simulink model "Model_GBXCluctchOpt_V5"  (R2024b)
settings: Solver=VariableStepAuto  StartTime=0.0  StopTime=552  RelTol=1e-5
undefined symbols (not defined in the file): Bdy_facCoG_C, Bdy_facTireFric_C, Bdy_lenRadiusWheel_C, Bdy_lenWheelBase_C, Bdy_lenZCoG_C, Bdy_mEquivalentJ_C, Bdy_mVeh_C, Bdy_vsqr2frc_C, Drv_kmh2gradtqDriver_C, Drv_kmh2tqDriver_C, Edr_pwr_LossMap_AXIS, Edr_pwrInverterLosses_MAP, Edr_pwrMachineLosses_MAP, Edr_rpm_InvLossMap_AXIS, Edr_rpm_MachLossMap_AXIS, Edr_rpm_MaxMinTq_AXIS, Edr_rpmMax_C, Edr_tq_MachLossMap_AXIS, Edr_tqEffMax_CUR, Env_facSlope_WLTC_CUR, Env_facSlopeBAB185_CUR, Env_facSlopeCrossCountry_CUR, Env_kmhDesBAB185_CUR, Env_kmhDesCrossCountry_CUR, Env_vVehDes_NEDC_kmh, Env_vVehDes_WLTC_kmh, Env_vVehTime_NEDC_s, Env_vVehTime_WLTC_s, Gbx_facGbxRatioRe_C, Ice_derfacLoadDecrease_MAP, Ice_derfacLoadIncrease_MAP, Ice_etaLam_CUR, Ice_facEtaCocMax_MAP, Ice_facFuelEnRich_MAP, Ice_KUMSRL_C, Ice_Lambda_AXIS, Ice_relLoad2relTqOptIgnLamOne_MAP, Ice_relLoad_AXIS, Ice_relLoad_LoadDyn_AXIS, Ice_relLoad_Max_CUR, Ice_relTq_AXIS, Ice_relTqInr2TqInr_C, Ice_relTqOptIgnLamOne2relLoad_MAP, Ice_rpm_AXIS, Ice_rpm_LoadDyn_AXIS, Ice_rpm_relLoadMax_AXIS, Ice_tqLossesIce_MAP, Pnt_capBat_C, Pnt_facSocBatOcv_AXIS, Pnt_facSocInit_C, Pnt_iBatChrgMax_C, Pnt_iBatDisChrgMax_C, Pnt_resBatInner_C, Pnt_uBatMax_C, Pnt_uBatMin_C, Pnt_uBatOcv_CUR, Vco_flgEdrExists_CFG, Vco_flgIceCluAlwClosed_CFG, Vco_flgIceExists_CFG
libraries: simulink x7, simulink_extras x6
(part 3 of 3)

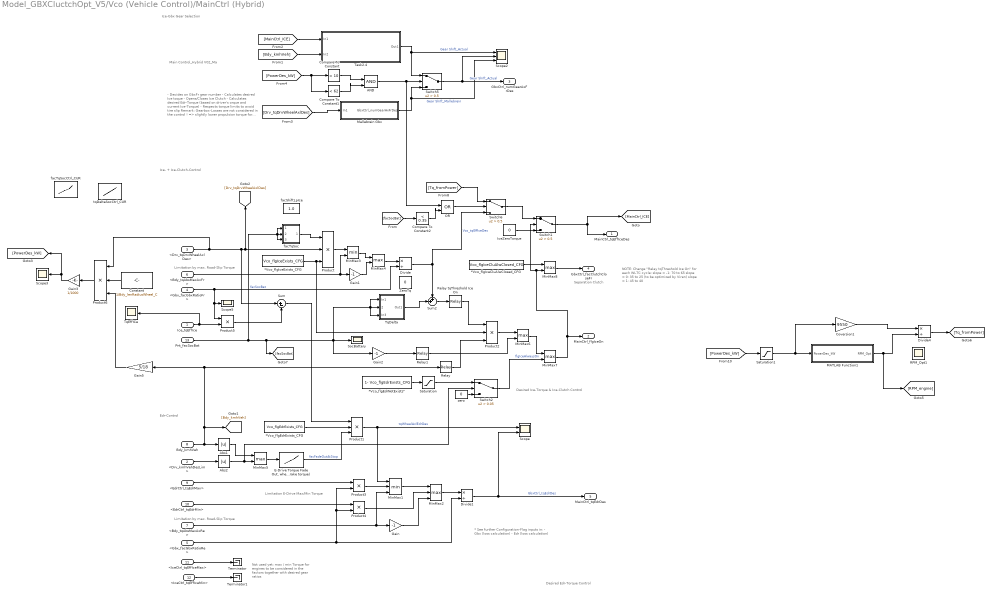
== system Model_GBXCluctchOpt_V5/Vco (Vehicle Control)/MainCtrl (Hybrid) ==
  note: Separation Clutch
  note: * See further Configuration-Flag inputs in:
      |    - Gbx (loss calculation)
      |    - Edr (loss calculation)
  note: Limitation E-Drive Max/Min Torque
  note: Not used yet:
      | max / min Torque for engines
      | to be considered in the factors
      | together with desired gear ratios
  note: Limitation by max. Road-Slip Torque
  note: Main Control_Hybrid V02_Ma
  note: - Decides on GbxFr gear number
      | - Calculates desired Ice toque
      | - Opens/Closes Ice Clutch
      | - Calculates desired Edr-Torque
      |   (based on driver's orque and current Ice-Torque)
      | - Respects torque limits to avoid tire slip
      |
      | Remark:
      | Gearbox-Losses are not considered in the control !
      | => slightly lower propulsion torque for Edr and Ice
      | => also in torque limitation
  note: Desired Ice-Torque & Ice-Clutch Control
  note: Desired Edr-Torque Control
  note: Limitation by max. Road-Slip Torque
  note: Edr-Control
  note: Ice- + Ice-Clutch-Control
  note: Ice-Gbx Gear Selection
  note: NOTE: Change "Relay tqThreshold Ice On" for each WLTC cycle:
      |
      | slope = -1: 70 to 65
      |
      | slope = 0: 35 to 25 (to be optimized by Viren)
      |
      | slope = 1: 45 to 40
  Ice_tqEffIce : Inport
  <Drv_kmhVehDesLim> : Inport  Port=2
  <Drv_tqDrvWheelAxlDes> : Inport  Port=3
  <Gbx_facGbxRatioFr> : Inport  Port=4
  <Gbx_facGbxRatioRe> : Inport  Port=5
  <Bdy_tqAbsMaxAxFr> : Inport  Port=6
  <Bdy_tqAbsMaxAxRe> : Inport  Port=7
  Bdy_kmhVeh : Inport  Port=8
  <EdrCtrl_tqEdrMax> : Inport  Port=9
  <EdrCtrl_tqEdrMin> : Inport  Port=10
  <IceCtrl_tqEffIceMax> : Inport  Port=11
  <IceCtrl_tqEffIceMin> : Inport  Port=12
  Pnt_facSocBat : Inport  Port=13
  *Vco_flgEdrExists_CFG : Constant  Value=Vco_flgEdrExists_CFG
  "*Vco_flgEdrNotExists\"" : Constant  Value=1- Vco_flgEdrExists_CFG
  *Vco_flgIceCluAlwClosed_CFG : Constant  Value=Vco_flgIceCluAlwClosed_CFG
  *Vco_flgIceExists_CFG : Constant  Value=Vco_flgIceExists_CFG
  AND : Logic  IconShape=distinctive  AllPortsSameDT=off  OutDataTypeStr=boolean
  Abs1 : Abs  ZeroCross=off  SaturateOnIntegerOverflow=off
  Abs2 : Abs  ZeroCross=off  SaturateOnIntegerOverflow=off
  Compare To Constant : simulink/Logic and Bit Operations/Compare To Constant  relop=>  const=10  OutDataTypeStr=boolean
  Compare To Constant1 : simulink/Logic and Bit Operations/Compare To Constant  relop=<  const=62  OutDataTypeStr=boolean
  Compare To Constant2 : simulink/Logic and Bit Operations/Compare To Constant  relop=<  const=0.35  OutDataTypeStr=boolean
  Constant : Constant  Value=1/Bdy_lenRadiusWheel_C
  Coversion1 : Gain  Gain=9550
  Divide : Product  Inputs=*/
  Divide1 : Product  Inputs=*/
  Divide4 : Product  Inputs=*/
  "E-Drive Torque Fade Out, when vehicle stops (To be harmonized with desired brake torque)" : Lookup_n-D  NumberOfTableDimensions=1  BreakpointsForDimension1=[-0.1 0 0.1 0.2]  Table="[ 0  1  1  1]"  InternalRulePriority=Speed  RndMeth=Simplest
  Gain : Gain  Gain=-1
  Gain1 : Gain  Gain=-1
  Gain2 : Gain  Gain=-1
  Gain3 : Gain  Gain=1/1000
  Gain5 : Gain  Gain=5/18
  IceZeroTorque : Constant  Value=0
  MATLAB Function1 : MATLAB Function  TreatAsAtomicUnit=on
  Mallebrein Gbx : Subsystem
  MinMax1 : MinMax  Inputs=3
  MinMax2 : MinMax  Function=max  Inputs=3  ZeroCross=off
  MinMax3 : MinMax  Inputs=2
  MinMax{4..8} (5 alike) : MinMax  Function=max  Inputs=2  ZeroCross=off
  OR : Logic  Operator=OR  IconShape=distinctive  AllPortsSameDT=off  OutDataTypeStr=boolean
  Product{,1..2,6} (4 alike) : Product  Inputs=3
  Product3 : Product
  Product4 : Product
  Product5 : Product
  RPM_Opt1 : Scope
  Relay : Relay  OnSwitchValue=30  OffSwitchValue=20
  Relay tqThreshold Ice On : Relay  OnSwitchValue=70  OffSwitchValue=65
  Relay1 : Relay  OnSwitchValue=-0.35  OffSwitchValue=-.38
  Saturation : Saturate  UpperLimit=1  LowerLimit=0
  Saturation1 : Saturate  UpperLimit=inf  LowerLimit=0
  Scope : Scope  NumInputPorts=2
  Scope2 : Scope  NumInputPorts=3
  Scope3 : Scope
  Scope5 : Scope
  SocBattery : Scope
  Sum : Sum  Inputs=|+-
  Sum2 : Sum  Inputs=++|
  Switch1 : Switch  Criteria=u2 > Threshold  Threshold=0.5  SaturateOnIntegerOverflow=off  InputSameDT=off
  Switch2 : Switch  Criteria=u2 > Threshold  Threshold=0.05  ZeroCross=off  SaturateOnIntegerOverflow=off  InputSameDT=off
  Switch5 : Switch  Criteria=u2 > Threshold  Threshold=0.5  SaturateOnIntegerOverflow=off  InputSameDT=off
  Switch6 : Switch  Criteria=u2 > Threshold  Threshold=0.5  SaturateOnIntegerOverflow=off  InputSameDT=off
  Task2.4 : Subsystem
  Terminator : Terminator
  Terminator1 : Terminator
  TqDelta : Subsystem
  TqEffICe : Scope
  ZeroTq : Constant  Value=0
  facShiftLpIce : Constant  Value=1.0
  facTqSoc : Subsystem
  facTqSocCtrl_CUR : Lookup_n-D  NumberOfTableDimensions=1  BreakpointsForDimension1="[0    0.1   0.2   0.3  0.4    0.6      0.7  0.8   0.9      1]"  Table="[1.4  1.3  1.2  1.1   1.05  0.95    0.9   0.8   0.65  0.5]"  ExtrapMethod=Clip  InternalRulePriority=Speed  RndMeth=Simplest
  tqDeltaSocCtrl_CUR : Lookup_n-D  NumberOfTableDimensions=1  BreakpointsForDimension1="[0    0.1   0.2   0.3  0.4  0.6  0.7  0.8   0.9    1]"  Table="[20  15    10     5     0    -5    -15    -30   -50  -70]"  ExtrapMethod=Clip  InternalRulePriority=Speed  RndMeth=Simplest
  zero : Constant  Value=0
  MainCtrl_tqEffIceDes : Outport
  MainCtrl_flgIceOn : Outport  Port=2
  GbxCtrl_numGearAxFrDes : Outport  Port=3
  GbxCtrl_facClutchCloseFr : Outport  Port=4
  MainCtrl_tqEdrDes : Outport  Port=5
  wires:
  Divide1/1 -> MainCtrl_tqEdrDes/1, Scope/2  "GbxCtrl_tqEdrDes"
  <Gbx_facGbxRatioFr>/1 -> Scope5/1, Product5/1, Divide/2
  <Gbx_facGbxRatioRe>/1 -> Divide1/2, Product4/2, Product3/2
  Product/1 -> MinMax3/1
  *Vco_flgIceExists_CFG/1 -> Product/3, Product2/2
  MinMax1/1 -> MinMax2/1
  Product1/1 -> MinMax1/1, Scope/1  "tqWheelAxlEdrDes"
  Gain/1 -> MinMax2/3
  MinMax2/1 -> Divide1/1
  MinMax4/1 -> Divide/1
  <Bdy_tqAbsMaxAxFr>/1 -> MinMax3/2, Gain1/1
  MinMax3/1 -> MinMax4/1
  Gain1/1 -> MinMax4/2
  Product3/1 -> MinMax1/2
  <EdrCtrl_tqEdrMax>/1 -> Product3/1
  Product4/1 -> MinMax2/2
  <EdrCtrl_tqEdrMin>/1 -> Product4/1
  <IceCtrl_tqEffIceMax>/1 -> Terminator/1
  <IceCtrl_tqEffIceMin>/1 -> Terminator1/1
  <Bdy_tqAbsMaxAxRe>/1 -> MinMax1/3, Gain/1
  <Drv_kmhVehDesLim>/1 -> Abs2/1
  Abs1/1 -> MinMax5/1
  Abs2/1 -> MinMax5/2, Switch2/2
  MinMax5/1 -> "E-Drive Torque Fade Out, when vehicle stops (To be harmonized with desired brake torque)"/1
  "E-Drive Torque Fade Out, when vehicle stops (To be harmonized with desired brake torque)"/1 -> Product1/3  "facFadeOutAtStop"
  IceZeroTorque/1 -> Switch1/3
  Sum/1 -> Product1/1
  Product5/1 -> Sum/2
  Ice_tqEffIce/1 -> TqEffICe/1, Product5/2
  MinMax7/1 -> Switch1/2, MinMax8/2, MainCtrl_flgIceOn/1
  *Vco_flgEdrExists_CFG/1 -> Product1/2
  Product2/1 -> MinMax6/1
  "*Vco_flgEdrNotExists\""/1 -> Saturation/1
  Switch2/1 -> MinMax7/2  "flgIceAlwaysOn"
  MinMax8/1 -> GbxCtrl_facClutchCloseFr/1
  *Vco_flgIceCluAlwClosed_CFG/1 -> MinMax8/1
  Saturation/1 -> Switch2/1
  zero/1 -> Switch2/3
  <Drv_tqDrvWheelAxlDes>/1 -> Product6/1, Product/2, [Drv_tqDrvWheelAxlDes], Sum/1
  Divide/1 -> Sum2/1, Switch6/3  "Vco_tqEffIceDes"
  Relay tqThreshold Ice On/1 -> Product2/1
  Sum2/1 -> Relay tqThreshold Ice On/1
  Pnt_facSocBat/1 -> [facSocBat], Gain2/1, TqDelta/3(In3), TqDelta/1(In1), TqDelta/2(Pnt_facSocBat), SocBattery/1, facTqSoc/1(Pnt_facSocBat), facTqSoc/2(In2), facTqSoc/3(In3)  "facSocBat"
  TqDelta/1(Out1) -> Sum2/2
  facTqSoc/1(Out1) -> Product/1
  Bdy_kmhVeh/1 -> Abs1/1, Gain5/1, Relay/1, [Bdy_kmhVeh]
  [Drv_tqDrvWheelAxlDes] -> Mallebrein Gbx/1(In1)
  [Bdy_kmhVeh] -> Task2.4/2(In2)
  Switch1/1 -> MainCtrl_tqEffIceDes/1, [MainCtrl_ICE]
  [MainCtrl_ICE] -> Task2.4/1(In1)
  Relay/1 -> Product2/3
  Gain2/1 -> Relay1/1
  Relay1/1 -> MinMax6/2
  MinMax6/1 -> MinMax7/1
  Product6/1 -> Gain3/1
  Constant/1 -> Product6/2
  Gain3/1 -> [PowerDes_kW], Scope3/1
  [PowerDes_kW] -> Compare To Constant1/1, Compare To Constant/1
  Compare To Constant/1 -> AND/1
  Compare To Constant1/1 -> AND/2
  Gain5/1 -> Product6/3
  ? -> RPM_Opt1/1
  Divide4/1 -> [Tq_fromPower]
  Coversion1/1 -> Divide4/1
  MATLAB Function1/1(RPM_Opt) -> [RPM_engine], Divide4/2
  [PowerDes_kW] -> Saturation1/1
  Mallebrein Gbx/1(GbxCtrl_numGearAxFrDes) -> Scope2/3, Switch5/3  "Gear Shift_Mallebrein"
  Saturation1/1 -> Coversion1/1, MATLAB Function1/1(PowerDes_kW)
  Switch6/1 -> Switch1/1
  [facSocBat] -> Compare To Constant2/1
  AND/1 -> Switch5/2, OR/1
  Compare To Constant2/1 -> OR/2
  OR/1 -> Switch6/2
  [Tq_fromPower] -> Switch6/1
  Task2.4/1(Out1) -> Switch5/1, Scope2/1  "Gear Shift_Actual"
  Switch5/1 -> Scope2/2, GbxCtrl_numGearAxFrDes/1  "Gear Shift_Actual"

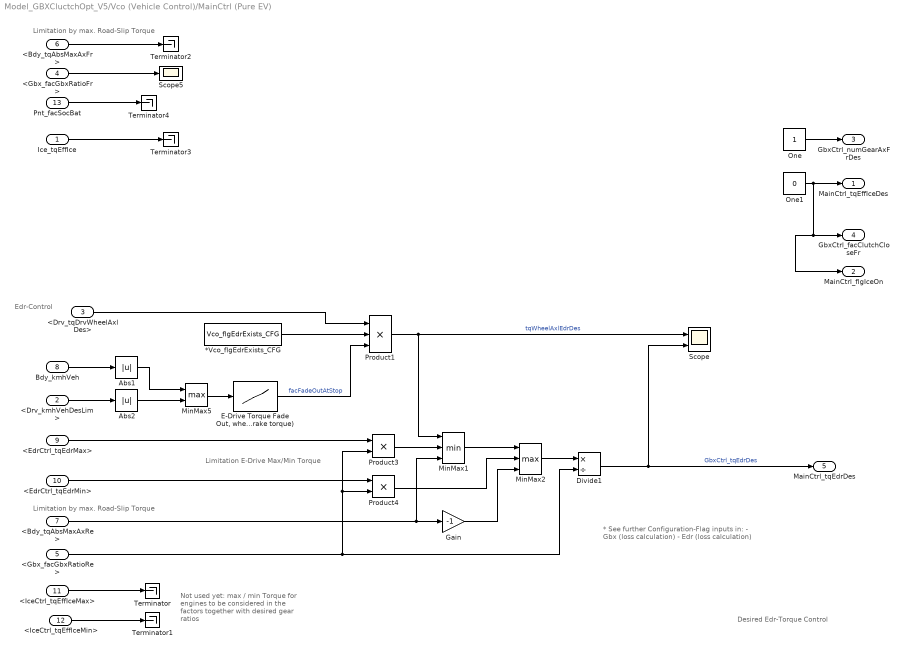
== system Model_GBXCluctchOpt_V5/Vco (Vehicle Control)/MainCtrl (Pure EV) ==
  note: * See further Configuration-Flag inputs in:
      |    - Gbx (loss calculation)
      |    - Edr (loss calculation)
  note: Limitation E-Drive Max/Min Torque
  note: Not used yet:
      | max / min Torque for engines
      | to be considered in the factors
      | together with desired gear ratios
  note: Limitation by max. Road-Slip Torque
  note: Desired Edr-Torque Control
  note: Limitation by max. Road-Slip Torque
  note: Edr-Control
  Ice_tqEffIce : Inport
  <Drv_kmhVehDesLim> : Inport  Port=2
  <Drv_tqDrvWheelAxlDes> : Inport  Port=3
  <Gbx_facGbxRatioFr> : Inport  Port=4
  <Gbx_facGbxRatioRe> : Inport  Port=5
  <Bdy_tqAbsMaxAxFr> : Inport  Port=6
  <Bdy_tqAbsMaxAxRe> : Inport  Port=7
  Bdy_kmhVeh : Inport  Port=8
  <EdrCtrl_tqEdrMax> : Inport  Port=9
  <EdrCtrl_tqEdrMin> : Inport  Port=10
  <IceCtrl_tqEffIceMax> : Inport  Port=11
  <IceCtrl_tqEffIceMin> : Inport  Port=12
  Pnt_facSocBat : Inport  Port=13
  *Vco_flgEdrExists_CFG : Constant  Value=Vco_flgEdrExists_CFG
  Abs1 : Abs  ZeroCross=off  SaturateOnIntegerOverflow=off
  Abs2 : Abs  ZeroCross=off  SaturateOnIntegerOverflow=off
  Divide1 : Product  Inputs=*/
  "E-Drive Torque Fade Out, when vehicle stops (To be harmonized with desired brake torque)" : Lookup_n-D  NumberOfTableDimensions=1  BreakpointsForDimension1=[-0.1 0.05 0.1 0.2]  Table="[ 0  0  1  1]"  InternalRulePriority=Speed  RndMeth=Simplest
  Gain : Gain  Gain=-1
  MinMax1 : MinMax  Inputs=3
  MinMax2 : MinMax  Function=max  Inputs=3  ZeroCross=off
  MinMax5 : MinMax  Function=max  Inputs=2  ZeroCross=off
  One : Constant
  One1 : Constant  Value=0
  Product1 : Product  Inputs=3
  Product3 : Product
  Product4 : Product
  Scope : Scope  NumInputPorts=2
  Scope5 : Scope
  Terminator{,1..4} (5 alike) : Terminator
  MainCtrl_tqEffIceDes : Outport
  MainCtrl_flgIceOn : Outport  Port=2
  GbxCtrl_numGearAxFrDes : Outport  Port=3
  GbxCtrl_facClutchCloseFr : Outport  Port=4
  MainCtrl_tqEdrDes : Outport  Port=5
  wires:
  Divide1/1 -> MainCtrl_tqEdrDes/1, Scope/2  "GbxCtrl_tqEdrDes"
  <Gbx_facGbxRatioFr>/1 -> Scope5/1
  <Gbx_facGbxRatioRe>/1 -> Divide1/2, Product4/2, Product3/2
  MinMax1/1 -> MinMax2/1
  Product1/1 -> MinMax1/1, Scope/1  "tqWheelAxlEdrDes"
  Gain/1 -> MinMax2/3
  MinMax2/1 -> Divide1/1
  Product3/1 -> MinMax1/2
  <EdrCtrl_tqEdrMax>/1 -> Product3/1
  Product4/1 -> MinMax2/2
  <EdrCtrl_tqEdrMin>/1 -> Product4/1
  <IceCtrl_tqEffIceMax>/1 -> Terminator/1
  <IceCtrl_tqEffIceMin>/1 -> Terminator1/1
  <Bdy_tqAbsMaxAxRe>/1 -> MinMax1/3, Gain/1
  <Drv_kmhVehDesLim>/1 -> Abs2/1
  Bdy_kmhVeh/1 -> Abs1/1
  Abs1/1 -> MinMax5/1
  Abs2/1 -> MinMax5/2
  MinMax5/1 -> "E-Drive Torque Fade Out, when vehicle stops (To be harmonized with desired brake torque)"/1
  "E-Drive Torque Fade Out, when vehicle stops (To be harmonized with desired brake torque)"/1 -> Product1/3  "facFadeOutAtStop"
  Ice_tqEffIce/1 -> Terminator3/1
  *Vco_flgEdrExists_CFG/1 -> Product1/2
  <Drv_tqDrvWheelAxlDes>/1 -> Product1/1
  <Bdy_tqAbsMaxAxFr>/1 -> Terminator2/1
  Pnt_facSocBat/1 -> Terminator4/1
  One/1 -> GbxCtrl_numGearAxFrDes/1
  One1/1 -> MainCtrl_flgIceOn/1, GbxCtrl_facClutchCloseFr/1, MainCtrl_tqEffIceDes/1

== system Model_GBXCluctchOpt_V5/Vco (Vehicle Control)/MainCtrl (Comb)/  Set has Prio   ==
  S : Inport
  R : Inport  Port=2
  Compare To Zero : simulink/Logic and Bit Operations/Compare To Zero  relop=<=  OutDataTypeStr=boolean
  Constant : Constant  Value=-1
  Integrator : Integrator  ExternalReset=level  InitialCondition=3  LimitOutput=on  UpperSaturationLimit=50  LowerSaturationLimit=0
  Logical Operator4 : Logic  AllPortsSameDT=off  OutDataTypeStr=boolean
  S-R Flip-Flop4 : simulink_extras/Flip Flops/S-R Flip-Flop  initial_condition=0
  Q : Outport
  wires:
  R/1 -> Logical Operator4/2
  S-R Flip-Flop4/1 -> Q/1
  S/1 -> S-R Flip-Flop4/1, Integrator/2
  Compare To Zero/1 -> Logical Operator4/1
  Logical Operator4/1 -> S-R Flip-Flop4/2
  Constant/1 -> Integrator/1
  Integrator/1 -> Compare To Zero/1

== system Model_GBXCluctchOpt_V5/Vco (Vehicle Control)/MainCtrl (Comb)/Gear Shift Improved ==
  note: 35...21
  note: 79...55
  note: 50...40
  note: Improved
  note: 18...13
  In 2 : Inport
  Gear 1 : Constant
  MinMax6 : MinMax  Function=max  Inputs=5
  Relay Gear 2 : Relay  OnSwitchValue=16  OffSwitchValue=13  OnOutputValue=2
  Relay Gear 3 : Relay  OnSwitchValue=26  OffSwitchValue=20  OnOutputValue=3
  Relay Gear 4 : Relay  OnSwitchValue=38  OffSwitchValue=30  OnOutputValue=4
  Relay Gear 5 : Relay  OnSwitchValue=50  OffSwitchValue=42  OnOutputValue=5
  2 : Outport
  wires:
  Relay Gear 3/1 -> MinMax6/3
  Relay Gear 4/1 -> MinMax6/4
  In 2/1 -> Relay Gear 5/1, Relay Gear 4/1, Relay Gear 3/1, Relay Gear 2/1
  Relay Gear 5/1 -> MinMax6/5
  Relay Gear 2/1 -> MinMax6/2
  Gear 1/1 -> MinMax6/1
  MinMax6/1 -> 2/1

== system Model_GBXCluctchOpt_V5/Vco (Vehicle Control)/MainCtrl (Comb)/Set has Prio ==
  S : Inport
  R : Inport  Port=2
  Compare To Zero : simulink/Logic and Bit Operations/Compare To Zero  relop=<=  OutDataTypeStr=boolean
  Constant : Constant  Value=-1
  Integrator : Integrator  ExternalReset=level  InitialCondition=3  LimitOutput=on  UpperSaturationLimit=50  LowerSaturationLimit=0
  Logical Operator4 : Logic  AllPortsSameDT=off  OutDataTypeStr=boolean
  S-R Flip-Flop4 : simulink_extras/Flip Flops/S-R Flip-Flop  initial_condition=0
  Scope9 : Scope  NumInputPorts=2
  Q : Outport
  wires:
  R/1 -> Logical Operator4/2
  S-R Flip-Flop4/1 -> Q/1
  S/1 -> S-R Flip-Flop4/1, Scope9/1, Integrator/2
  Compare To Zero/1 -> Scope9/2, Logical Operator4/1
  Logical Operator4/1 -> S-R Flip-Flop4/2
  Constant/1 -> Integrator/1
  Integrator/1 -> Compare To Zero/1

== system Model_GBXCluctchOpt_V5/Vco (Vehicle Control)/MainCtrl (Comb)/Set has Prio  ==
  S : Inport
  R : Inport  Port=2
  Compare To Zero : simulink/Logic and Bit Operations/Compare To Zero  relop=<=  OutDataTypeStr=boolean
  Constant : Constant  Value=-1
  Integrator : Integrator  ExternalReset=level  InitialCondition=3  LimitOutput=on  UpperSaturationLimit=50  LowerSaturationLimit=0
  Logical Operator4 : Logic  AllPortsSameDT=off  OutDataTypeStr=boolean
  S-R Flip-Flop4 : simulink_extras/Flip Flops/S-R Flip-Flop  initial_condition=0
  Q : Outport
  wires:
  R/1 -> Logical Operator4/2
  S-R Flip-Flop4/1 -> Q/1
  S/1 -> S-R Flip-Flop4/1, Integrator/2
  Compare To Zero/1 -> Logical Operator4/1
  Logical Operator4/1 -> S-R Flip-Flop4/2
  Constant/1 -> Integrator/1
  Integrator/1 -> Compare To Zero/1

== system Model_GBXCluctchOpt_V5/Vco (Vehicle Control)/MainCtrl (Comb)/Set has Prio   ==
  S : Inport
  R : Inport  Port=2
  Compare To Zero : simulink/Logic and Bit Operations/Compare To Zero  relop=<=  OutDataTypeStr=boolean
  Constant : Constant  Value=-1
  Integrator : Integrator  ExternalReset=level  InitialCondition=3  LimitOutput=on  UpperSaturationLimit=50  LowerSaturationLimit=0
  Logical Operator4 : Logic  AllPortsSameDT=off  OutDataTypeStr=boolean
  S-R Flip-Flop4 : simulink_extras/Flip Flops/S-R Flip-Flop  initial_condition=0
  Q : Outport
  wires:
  R/1 -> Logical Operator4/2
  S-R Flip-Flop4/1 -> Q/1
  S/1 -> S-R Flip-Flop4/1, Integrator/2
  Compare To Zero/1 -> Logical Operator4/1
  Logical Operator4/1 -> S-R Flip-Flop4/2
  Constant/1 -> Integrator/1
  Integrator/1 -> Compare To Zero/1

== system Model_GBXCluctchOpt_V5/Vco (Vehicle Control)/MainCtrl (Hybrid)/Mallebrein Gbx ==
  note: Bdy_kmhVeh
  note: default values are:
  note: unsym. Filter (fast up, slow down)
  note: only for propulsion
      | => in drag also shift down not realized
  note: 79..55
  note: 50..40
  note: 35..21
  note: 18..13
  note: Gear Selection
  In1 : Inport
  1-D Lookup Table : Lookup_n-D  NumberOfTableDimensions=1  BreakpointsForDimension1="[-10000 0  10000]"  Table="[-2000   0 200000]"  InternalRulePriority=Speed  RndMeth=Simplest
  Gear 1 : Constant
  Integrator : Integrator
  MinMax6 : MinMax  Function=max  Inputs=5
  Mux : Mux  Inputs=2
  Product6 : Product
  Relay Gear 2 : Relay  OnSwitchValue=18  OffSwitchValue=13  OnOutputValue=2
  Relay Gear 3 : Relay  OnSwitchValue=35  OffSwitchValue=21  OnOutputValue=3
  Relay Gear 4 : Relay  OnSwitchValue=50  OffSwitchValue=40  OnOutputValue=4
  Relay Gear 5 : Relay  OnSwitchValue=79  OffSwitchValue=55  OnOutputValue=5
  Scope2 : Scope
  Scope3 : Scope  NumInputPorts=2
  Scope4 : Scope
  Sum1 : Sum  Inputs=|+-
  facTqInfluence : Lookup_n-D  NumberOfTableDimensions=1  BreakpointsForDimension1="[0 10   500  1000   1500   2000   2500]"  Table="[1   1     0.9   0.8       0.7    0.6       0.5]"  ExtrapMethod=Clip  InternalRulePriority=Speed  RndMeth=Simplest
  GbxCtrl_numGearAxFrDes : Outport
  wires:
  Product6/1 -> Relay Gear 5/1, Relay Gear 4/1, Relay Gear 3/1, Relay Gear 2/1, Mux/1  "kmhModified"
  Sum1/1 -> 1-D Lookup Table/1
  MinMax6/1 -> GbxCtrl_numGearAxFrDes/1, Scope3/2, Scope2/1
  Integrator/1 -> facTqInfluence/1, Sum1/2
  In1/1 -> Scope4/1, Sum1/1
  Relay Gear 4/1 -> MinMax6/4
  Mux/1 -> Scope3/1
  Relay Gear 2/1 -> MinMax6/2
  facTqInfluence/1 -> Product6/2
  [Bdy_kmhVeh] -> Mux/2, Product6/1
  Gear 1/1 -> MinMax6/1
  Relay Gear 5/1 -> MinMax6/5
  Relay Gear 3/1 -> MinMax6/3
  1-D Lookup Table/1 -> Integrator/1

== system Model_GBXCluctchOpt_V5/Vco (Vehicle Control)/MainCtrl (Hybrid)/Task2.4 ==
  In1 : Inport
  In2 : Inport  Port=2
  1-D Lookup Table1 : Lookup_n-D  NumberOfTableDimensions=1  BreakpointsForDimension1=[50;120;130;160;180;190;230;240;250]  Table=[2000;2000;2000;2750;2750;3000;3000;2000;2000]  InternalRulePriority=Speed  RndMeth=Simplest
  1st Gear : Relay  OnSwitchValue=10  OffSwitchValue=8.5  OffOutputValue=6
  2*pi*wheelradius : Gain  Gain=2*3.14*Bdy_lenRadiusWheel_C
  2nd Gear : Relay  OnSwitchValue=8.5  OffSwitchValue=6  OnOutputValue=2  OffOutputValue=6
  3rd Gear : Relay  OnSwitchValue=6  OffSwitchValue=4.25  OnOutputValue=3  OffOutputValue=6
  4th Gear : Relay  OnSwitchValue=4.25  OffSwitchValue=3.1  OnOutputValue=4  OffOutputValue=6
  5th gear : Relay  OnSwitchValue=3.1  OffSwitchValue=1  OnOutputValue=5
  Constant : Constant  Value=0
  Constant1 : Constant  Value=-1
  Constant2 : Constant  Value=0
  Divide2 : Product  Inputs=*/
  Gain2 : Gain  Gain=60
  Min : MinMax  Inputs=5
  Scope : Scope  NumInputPorts=3
  Scope1 : Scope
  Switch : Switch  Criteria=u2 > Threshold  SaturateOnIntegerOverflow=off  InputSameDT=off
  Switch1 : Switch  Criteria=u2 ~= 0  SaturateOnIntegerOverflow=off  InputSameDT=off
  Switch3 : Switch  Criteria=u2 > Threshold  Threshold=10  SaturateOnIntegerOverflow=off  InputSameDT=off
  kmh2ms : Gain  Gain=5/18
  Out1 : Outport
  wires:
  2*pi*wheelradius/1 -> Divide2/1
  kmh2ms/1 -> Gain2/1
  1st Gear/1 -> Min/1
  In2/1 -> Scope/3, Switch1/2, Switch3/2, Switch3/1
  Switch3/1 -> kmh2ms/1
  Switch/1 -> Scope/2, 5th gear/1, 4th Gear/1, 3rd Gear/1, 2nd Gear/1, 1st Gear/1
  Gain2/1 -> Switch/2, Divide2/2
  Constant1/1 -> Switch3/3
  Divide2/1 -> Switch/1
  1-D Lookup Table1/1 -> 2*pi*wheelradius/1, Scope1/1
  Constant/1 -> Switch/3
  2nd Gear/1 -> Min/2
  In1/1 -> 1-D Lookup Table1/1
  4th Gear/1 -> Min/4
  3rd Gear/1 -> Min/3
  Min/1 -> Scope/1, Switch1/1
  5th gear/1 -> Min/5
  Switch1/1 -> Out1/1
  Constant2/1 -> Switch1/3

== system Model_GBXCluctchOpt_V5/Vco (Vehicle Control)/MainCtrl (Hybrid)/TqDelta ==
  In1 : Inport
  Pnt_facSocBat : Inport  Port=2
  In3 : Inport  Port=3
  Down_tqDeltaSocCtrl_CUR3 : Lookup_n-D  NumberOfTableDimensions=1  BreakpointsForDimension1=[0, 0.10, 0.20, 0.30, 0.40, 0.45, 0.48, 0.50, 0.52, 0.54, 0.55, 0.60, 0.70, 0.80, 1.0]  Table=[0, 0, 0, 0, 0, -10, -25, -45, -70, -100, -140, -180, -220, -260, -300]  ExtrapMethod=Clip  InternalRulePriority=Speed  RndMeth=Simplest
  From : From  TagVisibility=global
  MATLAB Function : MATLAB Function  TreatAsAtomicUnit=on
  Mild_Down_tqDeltaSocCtrl_CUR2 : Lookup_n-D  NumberOfTableDimensions=1  BreakpointsForDimension1=[0, 0.10, 0.20, 0.30, 0.40, 0.45, 0.50, 0.52, 0.54, 0.55, 0.60, 0.70, 0.80, 1.0]  Table=[0, 0, 0, 0, 0, -5, -15, -30, -50, -75, -100, -130, -160, -200]  ExtrapMethod=Clip  InternalRulePriority=Speed  RndMeth=Simplest
  Multiport Switch : MultiPortSwitch  DataPortOrder=Zero-based contiguous  zeroidx=on  SaturateOnIntegerOverflow=off  InputSameDT=off
  Up_tqDeltaSocCtrl_CUR1 : Lookup_n-D  NumberOfTableDimensions=1  BreakpointsForDimension1="[0    0.1   0.2   0.3  0.4  0.6  0.7  0.8   0.9    1]"  Table="[20  15    10     5     0    -5    -15    -30   -50  -70]"  ExtrapMethod=Clip  InternalRulePriority=Speed  RndMeth=Simplest
  Out1 : Outport
  wires:
  Pnt_facSocBat/1 -> Mild_Down_tqDeltaSocCtrl_CUR2/1
  Up_tqDeltaSocCtrl_CUR1/1 -> Multiport Switch/2
  Multiport Switch/1 -> Out1/1
  Mild_Down_tqDeltaSocCtrl_CUR2/1 -> Multiport Switch/3
  In3/1 -> Down_tqDeltaSocCtrl_CUR3/1
  Down_tqDeltaSocCtrl_CUR3/1 -> Multiport Switch/4
  In1/1 -> Up_tqDeltaSocCtrl_CUR1/1
  From/1 -> MATLAB Function/1(road_gradient)
  MATLAB Function/1(gradient_index) -> Multiport Switch/1

== system Model_GBXCluctchOpt_V5/Vco (Vehicle Control)/MainCtrl (Hybrid)/facTqSoc ==
  Pnt_facSocBat : Inport
  In2 : Inport  Port=2
  In3 : Inport  Port=3
  Down_facTqSocCtrl_CUR3 : Lookup_n-D  NumberOfTableDimensions=1  BreakpointsForDimension1=[0, 0.10, 0.20, 0.30, 0.40, 0.45, 0.48, 0.50, 0.52, 0.54, 0.55, 0.60, 0.70, 0.80, 1.0]  Table=[1.40, 1.30, 1.20, 1.10, 1.05, 1.00, 0.80, 0.60, 0.35, 0.15, 0.08, 0.03, 0.01, 0, 0]  ExtrapMethod=Clip  InternalRulePriority=Speed  RndMeth=Simplest
  From : From  TagVisibility=global
  MATLAB Function : MATLAB Function  TreatAsAtomicUnit=on
  Mild_Down_facTqSocCtrl_CUR2 : Lookup_n-D  NumberOfTableDimensions=1  BreakpointsForDimension1=[0, 0.10, 0.20, 0.30, 0.40, 0.45, 0.50, 0.52, 0.54, 0.55, 0.60, 0.70, 0.80, 1.0]  Table=[1.40, 1.30, 1.20, 1.10, 1.05, 1.00, 0.90, 0.70, 0.50, 0.40, 0.25, 0.15, 0.05, 0]  ExtrapMethod=Clip  InternalRulePriority=Speed  RndMeth=Simplest
  Multiport Switch : MultiPortSwitch  DataPortOrder=Zero-based contiguous  zeroidx=on  SaturateOnIntegerOverflow=off  InputSameDT=off
  Up_facTqSocCtrl_CUR1 : Lookup_n-D  NumberOfTableDimensions=1  BreakpointsForDimension1=[0;0.10000000000000001;0.20000000000000001;0.29999999999999999;0.40000000000000002;0.59999999999999998;0.69999999999999996;0.80000000000000004;0.90000000000000002;1]  Table=[1.4;1.3;1.2;1.1;1.05;0.95;0.9;0.8;0.65;0.5]  ExtrapMethod=Clip  InternalRulePriority=Speed  RndMeth=Simplest
  Out1 : Outport
  wires:
  In2/1 -> Mild_Down_facTqSocCtrl_CUR2/1
  Up_facTqSocCtrl_CUR1/1 -> Multiport Switch/2
  Multiport Switch/1 -> Out1/1
  In3/1 -> Down_facTqSocCtrl_CUR3/1
  MATLAB Function/1(gradient_index) -> Multiport Switch/1
  Pnt_facSocBat/1 -> Up_facTqSocCtrl_CUR1/1
  Down_facTqSocCtrl_CUR3/1 -> Multiport Switch/4
  From/1 -> MATLAB Function/1(road_gradient)
  Mild_Down_facTqSocCtrl_CUR2/1 -> Multiport Switch/3

== matlab function Model_GBXCluctchOpt_V5/Vco (Vehicle Control)/MainCtrl (Hybrid)/facTqSoc/MATLAB Function ==
  data: road_gradient input; gradient_index output
function gradient_index = fcn(road_gradient)
% Converts road gradient to lookup table index
% Inputs:  road_gradient (scalar double, range ±0.04)
% Outputs: gradient_index (uint8, values 0,1,2)

    if road_gradient > 0
        gradient_index = uint8(0);  % Uphill tables
    elseif road_gradient >= -0.02
        gradient_index = uint8(1);  % Flat/Mild Downhill tables
    else
        gradient_index = uint8(2);  % Steep Downhill tables
    end
end

== matlab function Model_GBXCluctchOpt_V5/Vco (Vehicle Control)/MainCtrl (Hybrid)/MATLAB Function1 ==
  data: PowerDes_kW input; RPM_Opt output
function RPM_Opt = fcn(PowerDes_kW)
% For be-specific range
tqMin = 120;    %Nm
tqMax = 200;    %Nm
RPM_Min = 1250;   %RPM
RPM_Max = 3000;   %RPM

if PowerDes_kW > 10 && PowerDes_kW < 25
    RPM_Opt = 1250;
elseif PowerDes_kW >= 25  && PowerDes_kW < 50
    RPM_Opt = 2250;
elseif PowerDes_kW >= 50 && PowerDes_kW <= 62 
    RPM_Opt = 3000;
else
    RPM_Opt = 2000;
end

== matlab function Model_GBXCluctchOpt_V5/Vco (Vehicle Control)/MainCtrl (Hybrid)/TqDelta/MATLAB Function ==
  data: road_gradient input; gradient_index output
function gradient_index = fcn(road_gradient)
% Converts road gradient to lookup table index
% Inputs:  road_gradient (scalar double, range ±0.04)
% Outputs: gradient_index (uint8, values 0,1,2)

    if road_gradient > 0
        gradient_index = uint8(0);  % Uphill tables
    elseif road_gradient >= -0.02
        gradient_index = uint8(1);  % Flat/Mild Downhill tables
    else
        gradient_index = uint8(2);  % Steep Downhill tables
    end
end
